simulink model "eval_discrete_model"  (R2026a)
settings: Solver=VariableStepAuto  StopTime=1000
undefined symbols (not defined in the file): ekf_param, perturbed_plant_param, r_param, random_seed
libraries: lib_plant x1
settings Model: Creator=alessandro-nardin  LastModifiedBy=alessandro-nardin

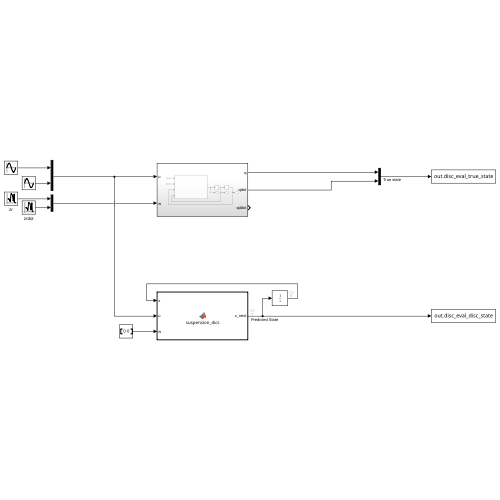
[thumbnail: Simulink's stored preview of the top-level diagram]
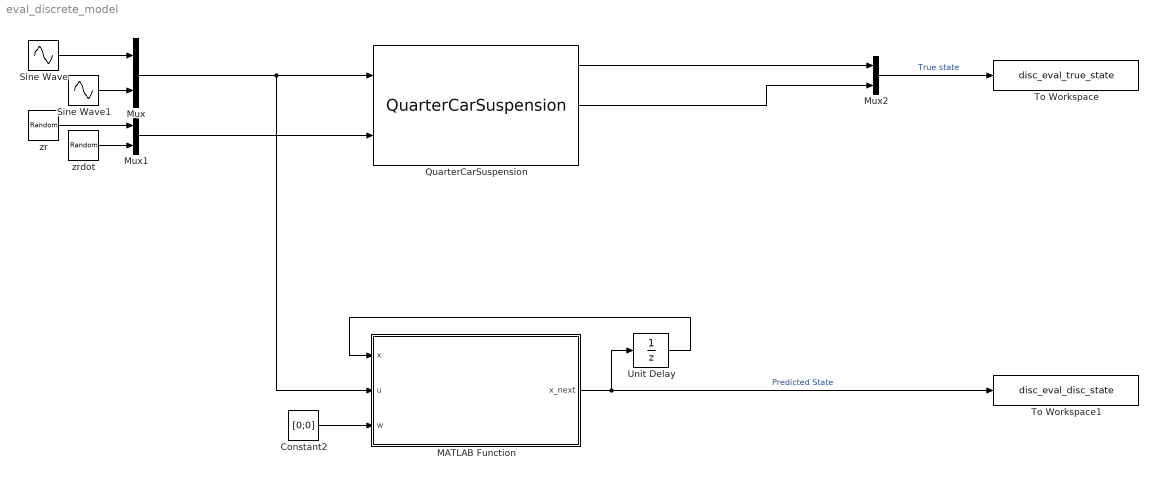
== system eval_discrete_model ==
  Constant2 : Constant  Value=[0;0]
  MATLAB Function : MATLAB Function  TreatAsAtomicUnit=on
  Mux : Mux  Inputs=2
  Mux1 : Mux  Inputs=2
  Mux2 : Mux  Inputs=2
  QuarterCarSuspension : lib_plant/QuarterCarSuspension  SystemSampleTime=-1  VariantActivationTime=update diagram  EmptyChoice=off  PassThrough=off  PassThroughVariantControl=(default)  EmptyChoiceVariantControl=(default)  AllowFlexibleInterface=on  Latency=0  AutoFrameSizeCalculation=off
      settings: SourceProductName=Lib Plant
  Sine Wave : Sin  Amplitude=1000  Frequency=0.5  SampleTime=0
  Sine Wave1 : Sin  Amplitude=1000  Frequency=0.5  SampleTime=0
  To Workspace : ToWorkspace  VariableName=disc_eval_true_state  SaveFormat=Timeseries  SampleTime=ekf_param.sample_t
  To Workspace1 : ToWorkspace  VariableName=disc_eval_disc_state  SaveFormat=Timeseries  SampleTime=ekf_param.sample_t
  Unit Delay : UnitDelay  InitialCondition=[1;0;0;0]  SampleTime=ekf_param.sample_t
  zr : RandomNumber  Variance=r_param.rz_var  Seed=random_seed+2  SampleTime=0
  zrdot : RandomNumber  Variance=r_param.rzdot_var  Seed=random_seed+3  SampleTime=0
  wires:
  MATLAB Function/1(x_next) -> To Workspace1/1, Unit Delay/1  "Predicted State"
  Mux1/1 -> QuarterCarSuspension/2
  Sine Wave/1 -> Mux/1
  Sine Wave1/1 -> Mux/2
  Mux/1 -> MATLAB Function/2(u), QuarterCarSuspension/1
  QuarterCarSuspension/1 -> Mux2/1
  QuarterCarSuspension/2 -> Mux2/2
  Unit Delay/1 -> MATLAB Function/1(x)
  zr/1 -> Mux1/1
  zrdot/1 -> Mux1/2
  Constant2/1 -> MATLAB Function/3(w)
  Mux2/1 -> To Workspace/1  "True state"

== matlab function eval_discrete_model/MATLAB Function ==
  settings: updateMethod=DISCRETE  sampleTime=ekf_param.sample_t
  data: x input; u input; x_next output size=[ 4 1 ]; w input; perturbed_plant_param parameter; ekf_param parameter
function x_next = suspension_dics( x, u, w, perturbed_plant_param, ekf_param)
x_next = suspension_f_dics_euler( x, u, w, perturbed_plant_param, ekf_param.sample_t);
